simulink model "if_multi_test_tmp"  (Simulink 8.3)
settings: Solver=VariableStepDiscrete  StartTime=0.0  StopTime=1  MaxStep=1  RelTol=1e-3
settings Model: Creator=arnaud  LastModifiedBy=hbourbou
settings DataIOCC: SaveFormat=Structure  SignalLoggingSaveFormat=Dataset
settings DebuggingCC: UnderspecifiedInitializationDetection=Simplified  MergeDetectMultiDrivingBlocksExec=error  FrameProcessingCompatibilityMsg=error  StateNameClashWarn=none
settings GRTTargetCC: CombineOutputUpdateFcns=on  GRTInterface=off

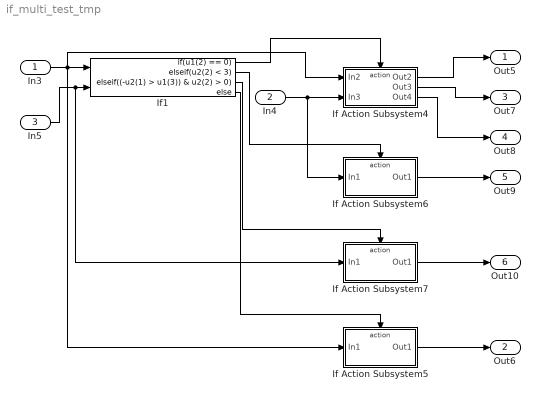
== system if_multi_test_tmp ==
  In3 : Inport  PortDimensions=3
  In4 : Inport  Port=2  OutDataTypeStr=boolean
  In5 : Inport  Port=3  PortDimensions=4
  If Action Subsystem4 : Subsystem  TreatAsAtomicUnit=on
  If Action Subsystem5 : Subsystem  TreatAsAtomicUnit=on
  If Action Subsystem6 : Subsystem  TreatAsAtomicUnit=on
  If Action Subsystem7 : Subsystem  TreatAsAtomicUnit=on
  If1 : If  NumInputs=2  IfExpression=u1(2) == 0  ElseIfExpressions=u2(2) < 3, (-u2(1) > u1(3)) & u2(2) > 0
  Out5 : Outport
  Out6 : Outport  Port=2
  Out7 : Outport  Port=3
  Out8 : Outport  Port=4
  Out9 : Outport  Port=5
  Out10 : Outport  Port=6
  wires:
  In3/1 -> If1/1, If Action Subsystem5/1(In1), If Action Subsystem4/1(In2)
  If1/1 -> If Action Subsystem4/Action
  If1/4 -> If Action Subsystem5/Action
  If Action Subsystem4/1(Out2) -> Out5/1
  If Action Subsystem5/1(Out1) -> Out6/1
  If Action Subsystem4/2(Out3) -> Out7/1
  In4/1 -> If Action Subsystem6/1(In1), If Action Subsystem4/2(In3)
  If Action Subsystem4/3(Out4) -> Out8/1
  If Action Subsystem6/1(Out1) -> Out9/1
  If Action Subsystem7/1(Out1) -> Out10/1
  If1/3 -> If Action Subsystem7/Action
  If1/2 -> If Action Subsystem6/Action
  In5/1 -> If Action Subsystem7/1(In1), If1/2

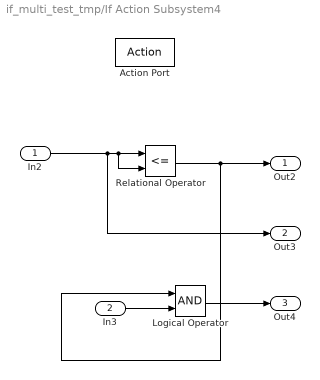
== system if_multi_test_tmp/If Action Subsystem4 ==
  In2 : Inport
  In3 : Inport  Port=2
  Action Port : ActionPort  ActionType=then
  Logical Operator : Logic  AllPortsSameDT=off  OutDataTypeStr=boolean
  Relational Operator : RelationalOperator  Operator=<=  OutDataTypeStr=boolean
  Out2 : Outport
  Out3 : Outport  Port=2
  Out4 : Outport  Port=3
  wires:
  In2/1 -> Relational Operator/1, Relational Operator/2, Out3/1
  Relational Operator/1 -> Logical Operator/1, Out2/1
  In3/1 -> Logical Operator/2
  Logical Operator/1 -> Out4/1

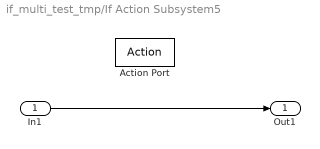
== system if_multi_test_tmp/If Action Subsystem5 ==
  In1 : Inport
  Action Port : ActionPort  ActionType=else
  Out1 : Outport
  wires:
  In1/1 -> Out1/1

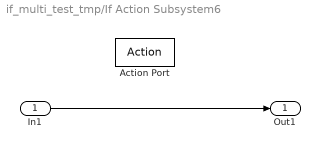
== system if_multi_test_tmp/If Action Subsystem6 ==
  In1 : Inport
  Action Port : ActionPort  ActionType=elseif
  Out1 : Outport
  wires:
  In1/1 -> Out1/1

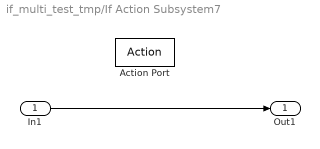
== system if_multi_test_tmp/If Action Subsystem7 ==
  In1 : Inport
  Action Port : ActionPort  ActionType=elseif
  Out1 : Outport
  wires:
  In1/1 -> Out1/1
